simulink model "Parcial"  (R2019a)
settings: Solver=VariableStepAuto  StartTime=0.0  StopTime=30  RelTol=1e-3
settings Model: Creator=jesus  LastModifiedBy=jesus

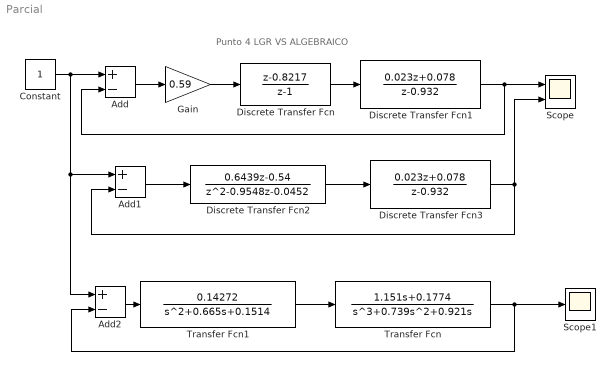
== system Parcial ==
  note: Punto 4 LGR VS ALGEBRAICO
  Add : Sum  Inputs=+-
  Add1 : Sum  Inputs=+-
  Add2 : Sum  Inputs=+-
  Constant : Constant
  Discrete Transfer Fcn : DiscreteTransferFcn  Numerator=[1 -0.8217]  Denominator=[1 -1]  SampleTime=0.05
  Discrete Transfer Fcn1 : DiscreteTransferFcn  Numerator=[0.023 0.078]  Denominator=[1 -0.932]  SampleTime=0.05
  Discrete Transfer Fcn2 : DiscreteTransferFcn  Numerator=[0.6439 -0.54]  Denominator=[1 -0.9548 -0.0452]  SampleTime=0.05
  Discrete Transfer Fcn3 : DiscreteTransferFcn  Numerator=[0.023 0.078]  Denominator=[1 -0.932]  SampleTime=0.05
  Gain : Gain  Gain=0.59
  Scope : Scope  NumInputPorts=2
  Scope1 : Scope
  Transfer Fcn : TransferFcn  Numerator=[1.151 0.1774]  Denominator=[1 0.739 0.921 0]
  Transfer Fcn1 : TransferFcn  Numerator=[0.14272]  Denominator=[1 0.665 0.1514]
  wires:
  Add/1 -> Gain/1
  Gain/1 -> Discrete Transfer Fcn/1
  Discrete Transfer Fcn/1 -> Discrete Transfer Fcn1/1
  Discrete Transfer Fcn1/1 -> Add/2, Scope/1
  Constant/1 -> Add2/1, Add1/1, Add/1
  Discrete Transfer Fcn3/1 -> Scope/2, Add1/2
  Add1/1 -> Discrete Transfer Fcn2/1
  Discrete Transfer Fcn2/1 -> Discrete Transfer Fcn3/1
  Transfer Fcn1/1 -> Transfer Fcn/1
  Add2/1 -> Transfer Fcn1/1
  Transfer Fcn/1 -> Add2/2, Scope1/1
